simulink model "working_kalman_old"  (R2025b)
settings: Solver=FixedStepDiscrete  StartTime=0.0  StopTime=+inf  FixedStep=simulink_Ts  RelTol=1e-3  EnableMultiTasking=on
InitFcn:
  | InitSensorFusion
values from neighbouring files (symbols this model uses):
  avg_order = 2    [InitSensorFusion_old.m]
  d = 0.15*sqrt(2)/2    [InitSensorFusion_old.m]
  friction_offset = 0.0001    [InitSensorFusion_old.m]
  friction_slope = 0.023e-3    (= 2.3e-05)    [InitSensorFusion_old.m]
  g = 9.81    [InitSensorFusion_old.m]
  Ic0 = Is0 + Iw0 - Iwg    [InitSensorFusion_old.m]
  ICM42_g = 9.8121    [InitSensorFusion_old.m]
  ICM42_gyr_offset = [-0.1319, -0.6878, 0.1737]    [InitSensorFusion_old.m]
  ICM42_params = params_1period    [InitSensorFusion_old.m]
  init_acc_bias = [0 0 0]'    [InitSensorFusion_old.m]
  init_P = P_initial    (= 10)    [InitSensorFusion_old.m]
  init_rot_quat = [0 0 0 1]'    [InitSensorFusion_old.m]
  kalman_Ts = 0.01    [InitSensorFusion_old.m]
  KV = 330    [InitSensorFusion_old.m]
  mc = mw + ms    (= 0.55)    [InitSensorFusion_old.m]
  sensor_Ts = 0.01    [InitSensorFusion_old.m]
  simulink_Ts = 0.01    [InitSensorFusion_old.m]
  stateInit = StateEnum.Initialization    [InitSensorFusion_old.m]
undefined symbols (not defined in the file or in its folder): init_time, StateEnum
libraries: mbedblockslib x24, stmnucleof7lib x5, nucleoutilitieslib x5, canmsglib x4, simulink x3, visionstatistics x2
(part 2 of 2)

== system working_kalman_old/MPU6050/Read sensing data/Subsystem2 ==
  In1 : Inport
  8g range : Gain  Gain=9.81275/4096
  Cast To Double : DataTypeConversion  OutDataTypeStr=double  SaturateOnIntegerOverflow=off  RndMeth=Floor
  Offset : Bias  SaturateOnIntegerOverflow=off
  Out1 : Outport
  wires:
  8g range/1 -> Offset/1  "Acc_Z"
  In1/1 -> Cast To Double/1
  Offset/1 -> Out1/1
  Cast To Double/1 -> 8g range/1

== system working_kalman_old/MPU6050/Read sensing data/Subsystem3 ==
  In1 : Inport
  8g range : Gain  Gain=9.81275/4096
  Cast To Double : DataTypeConversion  OutDataTypeStr=double  SaturateOnIntegerOverflow=off  RndMeth=Floor
  Offset : Bias  SaturateOnIntegerOverflow=off
  Out1 : Outport
  wires:
  8g range/1 -> Offset/1  "Acc_Z"
  In1/1 -> Cast To Double/1
  Offset/1 -> Out1/1
  Cast To Double/1 -> 8g range/1

== system working_kalman_old/MPU6050/Read sensing data/Subsystem4 ==
  In1 : Inport
  +-500 °/s range : Gain  Gain=1/65.5
  Cast To Double : DataTypeConversion  OutDataTypeStr=double  SaturateOnIntegerOverflow=off  RndMeth=Floor
  Offset : Bias  SaturateOnIntegerOverflow=off
  Out1 : Outport
  wires:
  Offset/1 -> Out1/1
  +-500 °/s range/1 -> Offset/1  "Acc_Z"
  Cast To Double/1 -> +-500 °/s range/1
  In1/1 -> Cast To Double/1

== system working_kalman_old/MPU6050/Read sensing data/Subsystem5 ==
  In1 : Inport
  +-500 °/s range : Gain  Gain=1/65.5
  Cast To Double : DataTypeConversion  OutDataTypeStr=double  SaturateOnIntegerOverflow=off  RndMeth=Floor
  Offset : Bias  SaturateOnIntegerOverflow=off
  Out1 : Outport
  wires:
  Offset/1 -> Out1/1
  +-500 °/s range/1 -> Offset/1  "Acc_Z"
  Cast To Double/1 -> +-500 °/s range/1
  In1/1 -> Cast To Double/1

== system working_kalman_old/MPU6050/Read sensing data/Subsystem6 ==
  In1 : Inport
  +-500 °/s range : Gain  Gain=1/65.5
  Cast To Double : DataTypeConversion  OutDataTypeStr=double  SaturateOnIntegerOverflow=off  RndMeth=Floor
  Offset : Bias  SaturateOnIntegerOverflow=off
  Out1 : Outport
  wires:
  Offset/1 -> Out1/1
  +-500 °/s range/1 -> Offset/1  "Acc_Z"
  Cast To Double/1 -> +-500 °/s range/1
  In1/1 -> Cast To Double/1

== matlab function working_kalman_old/Kalman sensor fusion ICM42/Quat2Euler ==
  settings: sampleTime=0.1
  data: Q input; EA output
function EA  = Quat2EulerAngles(Q)

% Q = normr(Q);

q0 = Q(1);
q1 = Q(2);
q2 = Q(3);
q3 = Q(4);

EA = [atan2d(-2*(q2.*q3 - q1.*q0), q0.^2 - q1.^2 - q2.^2 + q3.^2), ...
    asind(2*(q1.*q3 + q2.*q0)), ...
    atan2d(-2*(q1.*q2 - q3.*q0), q0.^2 + q1.^2 - q2.^2 - q3.^2)];

if ~isreal(EA)
    EA = real(EA);
end




end

== matlab function working_kalman_old/Kalman sensor fusion ICM42/Kalman Sensor Fusion for ICM42688-P ==
  settings: sampleTime=0.1
  data: data input; rot_quat_out output; acc_bias_out output; IMU_Fs input; Param input; g input; P_out output; rot_quat input; acc_bias input; P input; trc_P output; std_acc output; SIGMA_g output; criterion output
function [rot_quat_out, acc_bias_out, P_out, trc_P, std_acc, SIGMA_g, criterion]  = kalman_1period(data, IMU_Fs, Param, g, rot_quat, acc_bias, P)
%#codegen

% This function implements  the sensor fusion algorithm proposed in
% "Quaternion-Based Extended Kalman Filter for Determining Orientation by Inertial and Magnetic Sensing"
% by Angelo M. Sabatini, IEEE TRANSACTIONS ON BIOMEDICAL ENGINEERING, VOL. 53, NO. 7, JULY 2006
% &
% Estimating Three-Dimensional Orientation of Human Body Parts by Inertial/Magnetic Sensing
% by Angelo Maria Sabatini, Sensors 2011, 11, 1489-1525; doi:10.3390/s110201489

%%% This code originally implemented by
% Marco Caruso (Politecnico di Torino), marco.caruso@studenti.polito.it
% Date: 21/11/2019

% The ORIGINAL code was modified by Milad Nazarahari
% (nazaraha@ualberta.ca), during Ph.D. studies under supervision of Dr. H. Rouhani
% (hrouhani@ualberta.ca), University of Alberta, December 2020 as a part of
% a comparative/benchmarking study.

% The MATLAB code performs the operations of the ORIGINAL code except for:
% reference acceleration/magnetic field (Earth's magnetic field)
% was obtained from sensor readout during motionless perioed at the begining of the experiment
% & implementing adaptive parameter tuning (hard-switch) & accelerometer and
% magnetometer bias were added as states

%  --------------- INPUT ---------------
%%%% "data" including
% acc            = 1x3 (m/s^2)
% gyr            = 1x3 (rad/s)
% Fs             = sampling frequency of the IMU (Hz)
% QS             = 1x2 (s) motionless period at the begining of the trial

%%%% Params
% (1,1) SIGMA_g        = gyrsocope noise for process noise covariance matrix static
% (1,2) SIGMA_g        = gyrsocope noise for process noise covariance matrix dynamic
% (1,3) epsilon_g      = threshold for switching between (1,1) & (1,2)
% (1,4) stdBiasAcc_in  = 1x1 (m/s^2) initial value for Accelerometer bias covariance matrix
% (1,5) stdAcc         = accelerometer noise for measurement noise covariance matrix static
% (1,6) stdAcc         = accelerometer noise for measurement noise covariance matrix dynamic
% (1,7) epsilon_a      = threshold for switching between (1,5) & (1,6)

% --------------- OUTPUT ---------------
% rot_quat             = Nx4 [qx qy qz qw], the scalar part is at the END of the quaternion


%-------------NEEDS TO BE INITIALIAZED-----------------

% rot_quat = zeros(len, 4);
% P = Param(1)*eye(7); % initial error covariance matrix
% g = norm(mean(accel(QS(1)*IMU_Fs:QS(2)*IMU_Fs, :))); % gravitational acceleration


accel = data(1:3);
gyro = deg2rad(data(4:6));
% len = size(accel,1);
dt = 1/IMU_Fs;

quaternion = [rot_quat' acc_bias']';

% PROCESS NOISE
SIGMA_a = dt*Param(4)^2*eye(3);



    % Updating Gyro noise adaptively (Q)
    if norm(gyro) <= Param(3)
        std_gyr = Param(1);
    else
        std_gyr = Param(2);
    end

    % std_gyr = Param(1) - norm(gyro)*Param(2);

    SIGMA_g = std_gyr^2*eye(3);
    
    %%%%%%%%%%%%%%%%%%%%%%%%%%%%% PREDICTION %%%%%%%%%%%%%%%%%%%%%%%%%%%%%%%%
    wx = gyro(1); wy = gyro(2); wz = gyro(3);
    omega = 0.5*[0    wz -wy wx
        -wz    0     wx wy
        wy -wx    0    wz
        -wx -wy -wz  0];%skew symmetric

    % omega = 0.5*[0    -wz wy wx
    %     wz    0     -wx wy
    %     -wy wx    0    wz
    %     -wx -wy -wz  0];%skew symmetric


    Phi = [expm(omega*dt) zeros(4,3);
           zeros(3,4)     eye(3)     ];
    
    % Project the state ahead
    quaternion_ = Phi*quaternion;
    
    CSI = [[0 -quaternion(3) quaternion(2);
        quaternion(3) 0 -quaternion(1);
        -quaternion(2) quaternion(1) 0]+quaternion(4)*eye(3);...
        -quaternion(1:3)'];
    
    Q = [(dt/2)^2*CSI*SIGMA_g*CSI' zeros(4,3);
        zeros(3,4) SIGMA_a      ];
    
    % Compute the a priori covariance matrix
    P_= Phi*P*Phi'+Q;
    
    %%%%%%%%%%%%%%%%%%%%%%%%%%%%% UPDATE STEP %%%%%%%%%%%%%%%%%%%%%%%%%%%%%%%%
    q1 = quaternion_(1); q2 = quaternion_(2); q3 = quaternion_(3); q4 = quaternion_(4);
    
    % Linearize the measurement equation: Jacobian
    F = [2*g*[q3 -q4 q1 -q2
        q4 q3 q2 q1
        -q1 -q2 q3 q4],eye(3)];
        
    
    % Adapt the measurement covariance matrix
    C = [q1^2-q2^2-q3^2+q4^2 2*(q1*q2+q3*q4) 2*(q1*q3-q2*q4)
        2*(q1*q2-q3*q4) -q1^2+q2^2-q3^2+q4^2 2*(q2*q3+q1*q4)
        2*(q1*q3+q2*q4) 2*(q2*q3-q1*q4) -q1^2-q2^2+q3^2+q4^2];
    
    criterion = norm(accel' - C*[0;0;g] - quaternion_(5:7));
    criterion = norm(accel) - g;
    criterion = norm(accel - C*[0;0;g] - quaternion_(5:7));

    % Accelerometer
    if norm(accel - C*[0;0;g]) < Param(7) % (Eq 70 in 2011 paper)   - quaternion_(5:7)
    % if (norm(accel) - g) < Param(7)
        std_acc = Param(5);
    else
        std_acc = Param(6);
    end
    % std_acc = Param(5) + criterion*Param(6)/g;
    
    % Measurement covariance
    R = std_acc^2*eye(3);
    
    % Compute the Kalman Gain
    K = P_* F' * (F * P_ * F' + R)^-1;
    
    % Compute the a posteriori state estimate
    z = accel; % measurement vector
    z_predict = C*[0; 0; g]; %+ quaternion_(5:end);
    quaternion = quaternion_ + K*(z - z_predict);
    
    % Normalize the quaternion
    quaternion(1:4) = quaternion(1:4)/norm(quaternion(1:4));
    
    % Compute the a posteriori covariance matrix
    P_out = P_ - K*F*P_;
    
    rot_quat_out = quaternion(1:4);
    acc_bias_out = quaternion(5:7);
    
    trc_P = trace(P_out);

    
end

== matlab function working_kalman_old/MATLAB Function ==
  data: u input; mean output; last_mean input; N input; N output
function [mean, N] = running_mean(u, last_mean, N)

N = N + 1;

if(N>1)
    mean = 1/N*(last_mean*(N-1)+u);
else
    mean = u;
end

== matlab function working_kalman_old/Calibration and averaging/Subsystem2/MATLAB Function1 ==
  data: g_vector input; g_scalar output
function g_scalar = norm(g_vector)


g_scalar = norm(g_vector);

== matlab function working_kalman_old/Calibration and averaging/MATLAB Function1 ==
  data: u input size=[1, 6]; avg output size=[6, 1]; avg_w input size=[avg_order,6]; avg_w output; avg_order parameter
function [avg, avg_w] = mov_avg(u, avg_w, avg_order)


% avg_order = 4;

avg_w = [u; avg_w(1:avg_order - 1,:)];

avg = mean(avg_w)';

== matlab function working_kalman_old/State Machine/State Updates/MATLAB Function2 ==
  data: state input Enum: StateEnum size=1; button_pushed input; seconds_counter input; state output; time_elapsed input; time_when_elapsed input uint16; time_when_elapsed output; calibration_time parameter

function [state, time_when_elapsed] = updateState(state, button_pushed, seconds_counter, time_elapsed, time_when_elapsed, calibration_time)
%#codegen

    switch(state)
        
        case StateEnum.Initialization
            if(time_elapsed)
                state = StateEnum.Calibration;
                time_when_elapsed = seconds_counter + calibration_time;
            end

        case StateEnum.Calibration
            if(time_elapsed)
                state = StateEnum.Idle;
            end

        case StateEnum.Idle
            if(button_pushed)
                state = StateEnum.StartingMotors;
            end

        case StateEnum.StartingMotors
            state = StateEnum.Running;
        
        case StateEnum.Running
            if(button_pushed)
                state = StateEnum.StoppingMotors;
            end

        case StateEnum.StoppingMotors
            state = StateEnum.Idle;
        
        case StateEnum.Error
    end
end
